simulink model "SimPractice1"  (R2018a)
settings: Solver=ode45  StartTime=0.0  StopTime=5.0  RelTol=1e-9
undefined symbols (not defined in the file): F, k, m, r
settings Model: Creator=dirlak  LastModifiedBy=dirlak

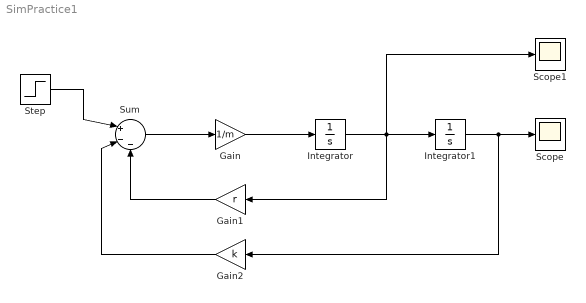
== system SimPractice1 ==
  Gain : Gain  Gain=1/m
  Gain1 : Gain  Gain=r
  Gain2 : Gain  Gain=k
  Integrator : Integrator
  Integrator1 : Integrator
  Scope : Scope
  Scope1 : Scope
  Step : Step  Time=0  After=F  SampleTime=0
  Sum : Sum  Inputs=|+--
  wires:
  Sum/1 -> Gain/1
  Gain/1 -> Integrator/1
  Integrator/1 -> Scope1/1, Gain1/1, Integrator1/1
  Integrator1/1 -> Gain2/1, Scope/1
  Step/1 -> Sum/1
  Gain1/1 -> Sum/3
  Gain2/1 -> Sum/2
